simulink model "motorPlate"  (R2019b)
settings: Solver=FixedStepAuto  StartTime=0.0  StopTime=100.0  FixedStep=0.001  RelTol=1e-3
values from neighbouring files (symbols this model uses):
  C_v = 16.5    [init.m]
  g = 9.81    [init.m]
  I_p = m_p*0.04^2/12    (= 0.00012)    [init.m]
  K = 11    [init.m]
  m_m = 0.118    [init.m]
  m_p = 0.9    [init.m]
  r = 0.17    [init.m]
undefined symbols (not defined in the file or in its folder): Continuous, I_0, plateLQRgain, Time, Ymp0
libraries: ctrlSharedLib x1
settings Model: Creator=chukh  LastModifiedBy=chukh

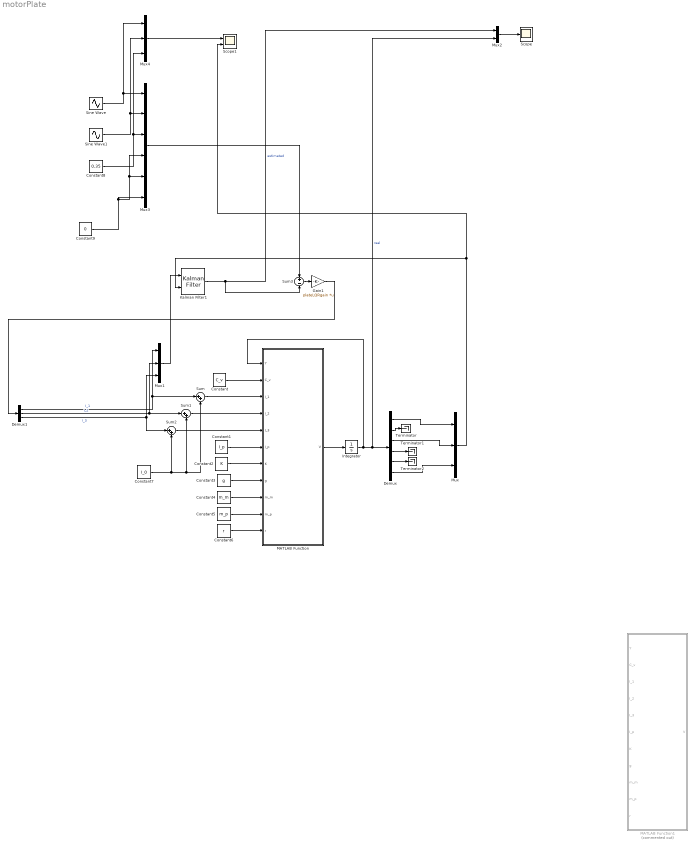
== system motorPlate ==
  Constant : Constant  Value=C_v
  Constant1 : Constant  Value=I_p
  Constant2 : Constant  Value=K
  Constant3 : Constant  Value=g
  Constant4 : Constant  Value=m_m
  Constant5 : Constant  Value=m_p
  Constant6 : Constant  Value=r
  Constant7 : Constant  Value=I_0
  Constant8 : Constant  Value=0.35
  Constant9 : Constant  Value=0
  Demux : Demux  Outputs=6
  Demux1 : Demux  Outputs=3
  Gain1 : Gain  Gain=plateLQRgain  Multiplication=Matrix(K*u)
  Integrator : Integrator  InitialCondition=Ymp0
  Kalman Filter1 : ctrlSharedLib/Kalman Filter  TimeDomain=Continuous-Time  UseCurrentEstimator=on  ModelSource=LTI State-Space Variable  ModelSourceVariable=plateSystem  A=0.95  B=1  C=1  D=0  NumberOfStates=1  NumberOfInputs=1  NumberOfOutputs=1  InitialEstimateSource=Dialog  X0=[0;0;0.32;0;0;0]  P0=10  UseK=off  UseGH=off  NumberOfProcessNoiseInputs=1  G=1  TimeInvariantG=on  H=0  TimeInvariantH=on  Q=0.05  TimeInvariantQ=on  R=1  TimeInvariantR=on  N=0  TimeInvariantN=on  AddInputPort=on  AddEnablePort=off  OutputEstimatedY=off  OutputP=off  Ts=-1
      settings: SourceProductBaseCode=CT
  MATLAB Function : MATLAB Function  TreatAsAtomicUnit=on
  MATLAB Function1 : MATLAB Function  Commented=on  TreatAsAtomicUnit=on
  Mux : Mux  Inputs=3
  Mux1 : Mux  Inputs=3
  Mux2 : Mux  Inputs=2
  Mux3 : Mux  Inputs=6
  Mux4 : Mux  Inputs=3
  Scope : Scope
  Scope1 : Scope  NumInputPorts=2
  Sine Wave : Sin  Amplitude=0.01  SampleTime=0
  Sine Wave1 : Sin  Amplitude=0.015  SampleTime=0
  Sum : Sum  Inputs=|++
  Sum1 : Sum  Inputs=|++
  Sum2 : Sum  Inputs=|++
  Sum3 : Sum  Inputs=+-
  Terminator : Terminator
  Terminator1 : Terminator
  Terminator2 : Terminator
  wires:
  Demux1/3 -> Sum2/1, Mux1/3  "I_3"
  Constant2/1 -> MATLAB Function/7(K)
  Constant6/1 -> MATLAB Function/11(r)
  Constant3/1 -> MATLAB Function/8(g)
  Constant5/1 -> MATLAB Function/10(m_p)
  Constant1/1 -> MATLAB Function/6(I_p)
  Constant4/1 -> MATLAB Function/9(m_m)
  Demux1/2 -> Sum1/1, Mux1/2  "I_2"
  Constant/1 -> MATLAB Function/2(C_v)
  Demux1/1 -> Mux1/1, Sum/1  "I_1"
  Integrator/1 -> MATLAB Function/1(Y), Mux2/2, Demux/1  "real"
  MATLAB Function/1(V) -> Integrator/1
  Sum2/1 -> MATLAB Function/5(I_3)
  Sum1/1 -> MATLAB Function/4(I_2)
  Sum/1 -> MATLAB Function/3(I_1)
  Constant7/1 -> Sum/2, Sum1/2, Sum2/2
  Demux/1 -> Mux/1
  Demux/3 -> Mux/2
  Demux/6 -> Mux/3
  Demux/2 -> Terminator/1
  Demux/4 -> Terminator1/1
  Demux/5 -> Terminator2/1
  Mux/1 -> Scope1/2, Kalman Filter1/2
  Mux1/1 -> Kalman Filter1/1
  Kalman Filter1/1 -> Sum3/2, Mux2/1  "estimated"
  Mux2/1 -> Scope/1
  Gain1/1 -> Demux1/1
  Constant9/1 -> Mux3/4, Mux3/5, Mux3/6
  Sine Wave/1 -> Mux4/1, Mux3/1
  Sine Wave1/1 -> Mux4/2, Mux3/2
  Constant8/1 -> Mux4/3, Mux3/3
  Mux3/1 -> Sum3/1
  Sum3/1 -> Gain1/1
  Mux4/1 -> Scope1/1

== matlab function motorPlate/MATLAB Function1 ==
  data: V output; Y input; C_v input; I_1 input; I_2 input; I_3 input; I_p input; K input; g input; m_m input; m_p input; r input
function V = motorPlateODElinear(Y,C_v,I_1,I_2,I_3,I_p,K,g,m_m,m_p,r)
%MOTORPLATEODELINEAR
%    V = MOTORPLATEODELINEAR(T,Y,C_V,I_1,I_2,I_3,I_P,K,G,M_M,M_P,R)

%    This function was generated by the Symbolic Math Toolbox version 8.4.
%    25-May-2021 06:21:31

%matrix([[omega_2f], [omega_1f], [dz_Cf], [theta_1f], [theta_2f], [z_Cf]])
t2 = I_p.*2.0;
t3 = Y(1);
t4 = Y(2);
t5 = Y(3);
t6 = r.^2;
t7 = I_2.*K;
t8 = I_3.*K;
t9 = sqrt(3.0);
t10 = -t7;
t11 = -t8;
t12 = m_m.*t6.*3.0;
t13 = t2+t12;
t14 = 1.0./t13;
V = [r.*t14.*(t7+t8-I_1.*K.*2.0-C_v.*r.*t3.*3.0);-r.*t14.*(t8.*t9+t9.*t10+C_v.*r.*t4.*3.0);(t7+t8-C_v.*t5.*3.0-g.*m_m.*3.0-g.*m_p+I_1.*K)./(m_m.*3.0+m_p);t4;t3;t5];

== matlab function motorPlate/MATLAB Function ==
  data: V output; Y input; C_v input; I_1 input; I_2 input; I_3 input; I_p input; K input; g input; m_m input; m_p input; r input
function V = motorPlateODE(Y,C_v,I_1,I_2,I_3,I_p,K,g,m_m,m_p,r)
%MOTORPLATEODE
%    V = MOTORPLATEODE(Y,C_v,I_1,I_2,I_3,I_p,K,g,m_m,m_p,r)

%    This function was generated by the Symbolic Math Toolbox version 8.4.
%    18-May-2021 19:45:09

%matrix([[theta_1f], [omega_1f], [theta_2f], [omega_2f], [dz_Cf], [z_Cf]])
t2 = I_p.^2;
t3 = Y(1);
t4 = Y(2);
t5 = Y(3);
t6 = Y(4);
t7 = Y(5);
t8 = m_m.^2;
t9 = r.^2;
t10 = r.^3;
t19 = sqrt(3.0);
t11 = t9.^2;
t12 = cos(t3);
t13 = cos(t5);
t14 = sin(t3);
t15 = sin(t5);
t16 = t2.*4.0;
t17 = t4.^2;
t18 = t6.^2;
t20 = t12.^2;
t21 = t12.^3;
t22 = t13.^2;
t23 = t13.^3;
t25 = t14.^2;
t26 = t15.^2;
t24 = t22.^2;
t27 = I_p.*m_m.*t9.*t22.*6.0;
t29 = I_p.*m_m.*t9.*t25.*t26.*6.0;
t28 = t20.*t27;
t30 = t8.*t11.*t20.*t24.*9.0;
t31 = t16+t27+t28+t29+t30;
t32 = 1.0./t31;
V = [t4;t32.*(t12.*t14.*t17.*t27+t12.*t14.*t18.*t27+t8.*t11.*t12.*t14.*t17.*t24.*9.0+t8.*t11.*t12.*t14.*t18.*t24.*9.0-C_v.*I_p.*t4.*t9.*t20.*t22.*6.0-C_v.*m_m.*t4.*t11.*t20.*t24.*9.0+I_2.*I_p.*K.*r.*t12.*t13.*t19.*2.0-I_3.*I_p.*K.*r.*t12.*t13.*t19.*2.0+I_2.*K.*m_m.*t10.*t12.*t19.*t23.*3.0-I_3.*K.*m_m.*t10.*t12.*t19.*t23.*3.0+t4.*t6.*t8.*t11.*t15.*t20.*t23.*1.8e+1+t8.*t11.*t12.*t14.*t18.*t22.*t26.*1.8e+1-t8.*t11.*t14.*t18.*t21.*t22.*t26.*9.0-t8.*t11.*t12.*t14.^3.*t18.*t22.*t26.*9.0-t4.*t6.*t8.*t11.*t13.*t15.^3.*t20.*t25.*9.0+C_v.*I_p.*t6.*t9.*t12.*t13.*t14.*t15.*6.0-I_1.*K.*m_m.*t10.*t12.*t14.*t15.*t22.*6.0+I_2.*K.*m_m.*t10.*t12.*t14.*t15.*t22.*3.0+I_3.*K.*m_m.*t10.*t12.*t14.*t15.*t22.*3.0+I_p.*m_m.*t4.*t6.*t9.*t13.*t15.*t20.*1.2e+1+t4.*t6.*t8.*t11.*t13.*t15.*t20.*t25.*9.0-t4.*t6.*t8.*t11.*t15.*t20.*t23.*t25.*9.0);t6;-r.*t32.*(I_1.*I_p.*K.*t13.*4.0-I_2.*I_p.*K.*t13.*2.0-I_3.*I_p.*K.*t13.*2.0+C_v.*I_p.*r.*t6.*t22.*6.0-t8.*t10.*t15.*t18.*t20.*t23.*1.8e+1+t8.*t10.*t15.*t18.*t20.^2.*t23.*9.0+I_2.*I_p.*K.*t14.*t15.*t19.*2.0-I_3.*I_p.*K.*t14.*t15.*t19.*2.0+C_v.*I_p.*r.*t6.*t25.*t26.*6.0+I_1.*K.*m_m.*t9.*t20.*t23.*6.0-I_2.*K.*m_m.*t9.*t20.*t23.*3.0-I_3.*K.*m_m.*t9.*t20.*t23.*3.0+C_v.*m_m.*t6.*t10.*t20.*t24.*9.0-I_p.*m_m.*r.*t13.*t15.*t18.*1.2e+1-I_p.*m_m.*r.*t4.*t6.*t12.*t14.*6.0+I_p.*m_m.*r.*t13.*t15.*t18.*t20.*6.0+I_p.*m_m.*r.*t13.*t15.*t17.*t25.*6.0+I_p.*m_m.*r.*t13.*t15.*t18.*t25.*1.2e+1-t4.*t6.*t8.*t10.*t14.*t21.*t22.*9.0+t4.*t6.*t8.*t10.*t14.*t21.*t24.*9.0+t8.*t10.*t15.*t18.*t20.*t23.*t25.*9.0-C_v.*I_p.*r.*t4.*t12.*t13.*t14.*t15.*6.0+I_p.*m_m.*r.*t4.*t6.*t12.*t14.*t22.*6.0+I_p.*m_m.*r.*t4.*t6.*t12.*t14.*t26.*1.8e+1+t4.*t6.*t8.*t10.*t14.*t21.*t22.*t26.*9.0);-(C_v.*t7.*3.0+g.*m_m.*3.0+g.*m_p-I_1.*K-I_2.*K-I_3.*K)./(m_m.*3.0+m_p);t7];
end
